simulink model "Modele_thermique"  (R2019b)
settings: Solver=FixedStepAuto  StartTime=0.0  StopTime=10.0  FixedStep=.01  RelTol=1e-3
values from neighbouring files (symbols this model uses):
  g = 9.81    [init.m]
  MOT = CBR    [init.m]
  passage_rapport = [1 2 3 4 5 6]    [init.m]
  rapport_max = 3    [init.m]
  ROUE = R13H    [init.m]
  t_passage = 0.1    [init.m]
  v_passage = [0 62.7 80.5 95 107.9 118.3]/3.6    [init.m]
undefined symbols (not defined in the file or in its folder): AERO, TRANS, VEH
libraries: simulink x1
settings Model: Creator=guillaume  LastModifiedBy=guillaume

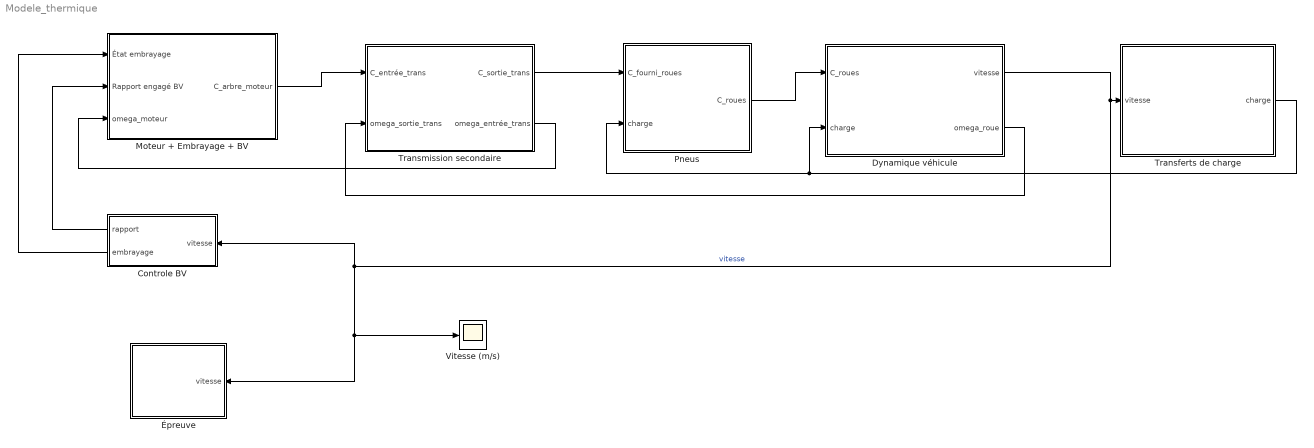
== system Modele_thermique ==
  Controle BV : Subsystem
  Dynamique véhicule : Subsystem
  Moteur + Embrayage + BV : Subsystem
  Pneus : Subsystem
  Transferts de charge : Subsystem
  Transmission secondaire : Subsystem
  Vitesse (m/s) : Scope
  Épreuve : Subsystem
  wires:
  Moteur + Embrayage + BV/1(C_arbre_moteur) -> Transmission secondaire/1(C_entrée_trans)
  Transmission secondaire/1(C_sortie_trans) -> Pneus/1(C_fourni_roues)
  Pneus/1(C_roues) -> Dynamique véhicule/1(C_roues)
  Transferts de charge/1(charge) -> Dynamique véhicule/2(charge), Pneus/2(charge)
  Dynamique véhicule/2(omega_roue) -> Transmission secondaire/2(omega_sortie_trans)
  Transmission secondaire/2(omega_entrée_trans) -> Moteur + Embrayage + BV/3(omega_moteur)
  Controle BV/1(rapport) -> Moteur + Embrayage + BV/2(Rapport engagé BV)
  Controle BV/2(embrayage) -> Moteur + Embrayage + BV/1("État embrayage ")
  Dynamique véhicule/1(vitesse) -> Controle BV/1(vitesse), Vitesse (m/s)/1, Épreuve/1(vitesse), Transferts de charge/1(vitesse)  "vitesse"

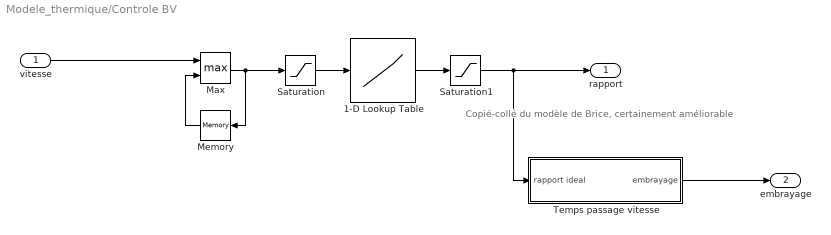
== system Modele_thermique/Controle BV ==
  note: Copié-collé du modèle de Brice, certainement améliorable
  vitesse : Inport
  1-D Lookup Table : Lookup_n-D  NumberOfTableDimensions=1  BreakpointsForDimension1=v_passage  IndexSearchMethod=Linear search  Table=passage_rapport  InterpMethod=Flat  DiagnosticForOutOfRangeInput=Warning  InternalRulePriority=Speed  OutMax=[3]  OutDataTypeStr=Inherit: Inherit from 'Table data'  RndMeth=Simplest  InputSameDT=on
  Max : MinMax  Function=max  Inputs=2
  Memory : Memory
  Saturation : Saturate  UpperLimit=inf  LowerLimit=0
  Saturation1 : Saturate  UpperLimit=rapport_max  LowerLimit=1
  "Temps passage vitesse " : Subsystem
  rapport : Outport
  embrayage : Outport  Port=2
  wires:
  vitesse/1 -> Max/1
  Max/1 -> Saturation/1, Memory/1
  Memory/1 -> Max/2
  Saturation/1 -> 1-D Lookup Table/1
  1-D Lookup Table/1 -> Saturation1/1
  "Temps passage vitesse "/1(embrayage) -> embrayage/1
  Saturation1/1 -> "Temps passage vitesse "/1(rapport ideal), rapport/1

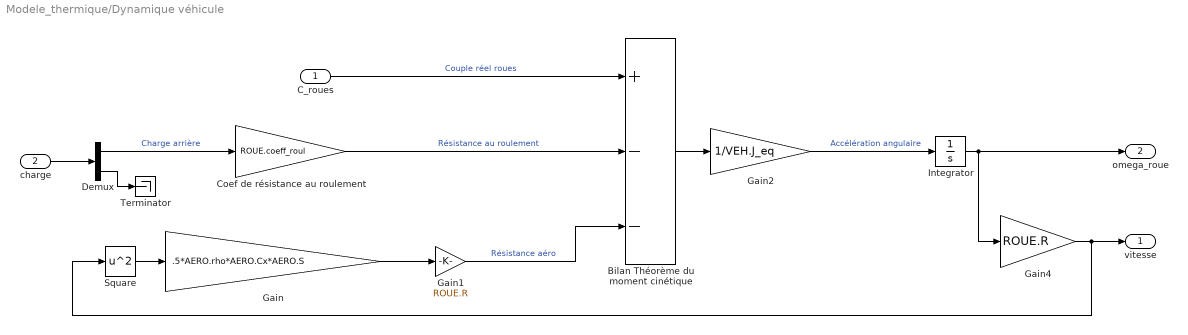
== system Modele_thermique/Dynamique véhicule ==
  C_roues : Inport
  charge : Inport  Port=2
  Bilan Théorème du moment cinétique : Sum  Inputs=+--
  Coef de résistance au roulement : Gain  Gain=ROUE.coeff_roul
  Demux : Demux  Outputs=2
  Gain : Gain  Gain=.5*AERO.rho*AERO.Cx*AERO.S
  Gain1 : Gain  Gain=ROUE.R
  Gain2 : Gain  Gain=1/VEH.J_eq
  Gain4 : Gain  Gain=ROUE.R
  Integrator : Integrator
  Square : Math  Operator=square  SignedPower=off  SaturateOnIntegerOverflow=on
  Terminator : Terminator
  vitesse : Outport
  omega_roue : Outport  Port=2
  wires:
  C_roues/1 -> Bilan Théorème du moment cinétique/1  "Couple réel roues"
  charge/1 -> Demux/1
  Demux/1 -> Coef de résistance au roulement/1  "Charge arrière"
  Coef de résistance au roulement/1 -> Bilan Théorème du moment cinétique/2  "Résistance au roulement"
  Square/1 -> Gain/1
  Gain/1 -> Gain1/1
  Gain1/1 -> Bilan Théorème du moment cinétique/3  "Résistance aéro"
  Bilan Théorème du moment cinétique/1 -> Gain2/1
  Gain2/1 -> Integrator/1  "Accélération angulaire"
  Integrator/1 -> omega_roue/1, Gain4/1
  Demux/2 -> Terminator/1
  Gain4/1 -> Square/1, vitesse/1

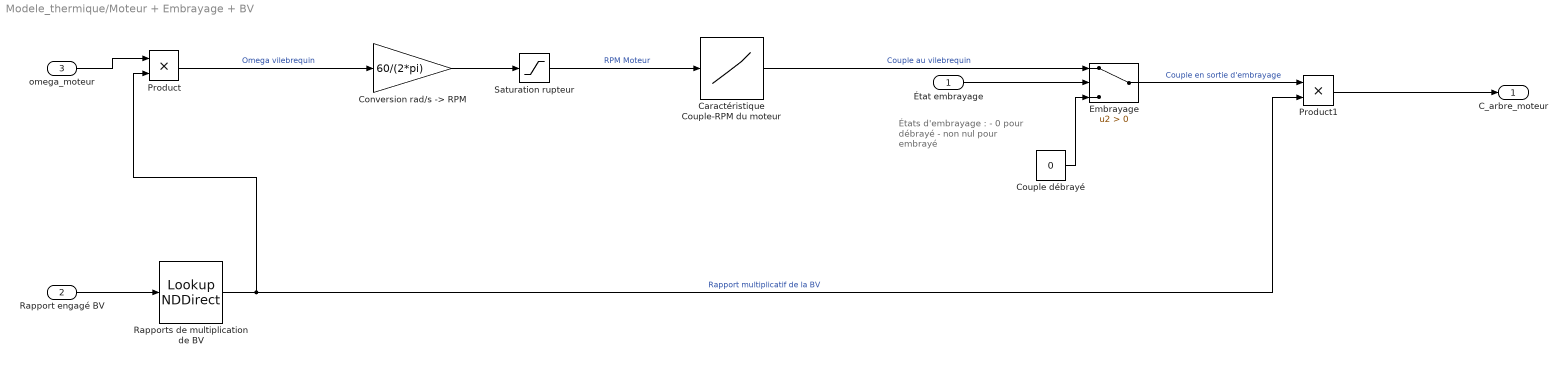
== system Modele_thermique/Moteur + Embrayage + BV ==
  note: États d'embrayage :
      | - 0 pour débrayé
      | - non nul pour embrayé
  "État embrayage " : Inport
  Rapport engagé BV : Inport  Port=2
  omega_moteur : Inport  Port=3
  Caractéristique Couple-RPM du moteur : Lookup_n-D  NumberOfTableDimensions=1  BreakpointsForDimension1=MOT.couple_RPM  Table=MOT.couple  InternalRulePriority=Speed  RndMeth=Simplest  InputSameDT=on
  "Conversion rad/s -> RPM" : Gain  Gain=60/(2*pi)
  Couple débrayé : Constant  Value=0
  Embrayage : Switch  Criteria=u2 > Threshold
  Product : Product
  Product1 : Product
  Rapports de multiplication de BV : LookupNDDirect  NumberOfTableDimensions=1  Table=[0 1./MOT.BV_rapports]  DiagnosticForOutOfRangeInput=Error
  Saturation rupteur : Saturate  UpperLimit=MOT.RPM_rupteur  LowerLimit=MOT.RPM_patinage
  C_arbre_moteur : Outport
  wires:
  Saturation rupteur/1 -> Caractéristique Couple-RPM du moteur/1  "RPM Moteur"
  Caractéristique Couple-RPM du moteur/1 -> Embrayage/1  "Couple au vilebrequin"
  Couple débrayé/1 -> Embrayage/3
  "État embrayage "/1 -> Embrayage/2
  Rapport engagé BV/1 -> Rapports de multiplication de BV/1
  Rapports de multiplication de BV/1 -> Product1/2, Product/2  "Rapport multiplicatif de la BV"
  Embrayage/1 -> Product1/1  "Couple en sortie d'embrayage"
  Product1/1 -> C_arbre_moteur/1
  "Conversion rad/s -> RPM"/1 -> Saturation rupteur/1
  Product/1 -> "Conversion rad/s -> RPM"/1  "Omega vilebrequin"
  omega_moteur/1 -> Product/1

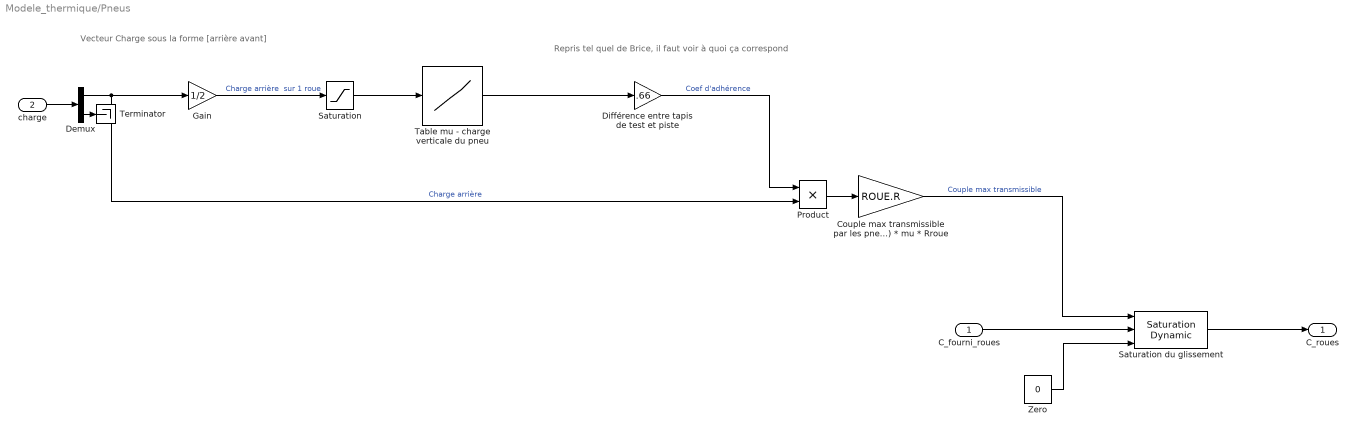
== system Modele_thermique/Pneus ==
  note: Repris tel quel de Brice,
      | il faut voir à quoi ça correspond
  note: Vecteur Charge sous la forme [arrière avant]
  C_fourni_roues : Inport
  charge : Inport  Port=2
  Couple max transmissible par les pneu chargés (2) * mu * Rroue : Gain  Gain=ROUE.R
  Demux : Demux  Outputs=2
  Différence entre tapis de test et piste : Gain  Gain=.66
  Gain : Gain  Gain=1/2
  Product : Product
  Saturation : Saturate  UpperLimit=ROUE.mupneu(1, end)  LowerLimit=ROUE.mupneu(1,1)
  Saturation du glissement : simulink/Discontinuities/Saturation Dynamic  OutMin=[0]  OutMax=[]  OutDataTypeStr=Inherit: Same as second input  OutDataType=fixdt(1, 16)  OutScaling=2^-10  DoSatur=off
  Table mu - charge verticale du pneu : Lookup_n-D  NumberOfTableDimensions=1  BreakpointsForDimension1=ROUE.mupneu(1,:)  Table=ROUE.mupneu(2,:)  DiagnosticForOutOfRangeInput=Error  InternalRulePriority=Speed  RndMeth=Simplest  InputSameDT=on
  Terminator : Terminator
  Zero : Constant  Value=0  OutDataTypeStr=Inherit: Inherit via back propagation
  C_roues : Outport
  wires:
  Saturation du glissement/1 -> C_roues/1
  Couple max transmissible par les pneu chargés (2) * mu * Rroue/1 -> Saturation du glissement/1  "Couple max transmissible"
  C_fourni_roues/1 -> Saturation du glissement/2
  charge/1 -> Demux/1
  Demux/1 -> Gain/1, Product/2  "Charge arrière"
  Table mu - charge verticale du pneu/1 -> Différence entre tapis de test et piste/1
  Différence entre tapis de test et piste/1 -> Product/1  "Coef d'adhérence"
  Product/1 -> Couple max transmissible par les pneu chargés (2) * mu * Rroue/1
  Gain/1 -> Saturation/1  "Charge arrière  sur 1 roue"
  Saturation/1 -> Table mu - charge verticale du pneu/1
  Demux/2 -> Terminator/1
  Zero/1 -> Saturation du glissement/3

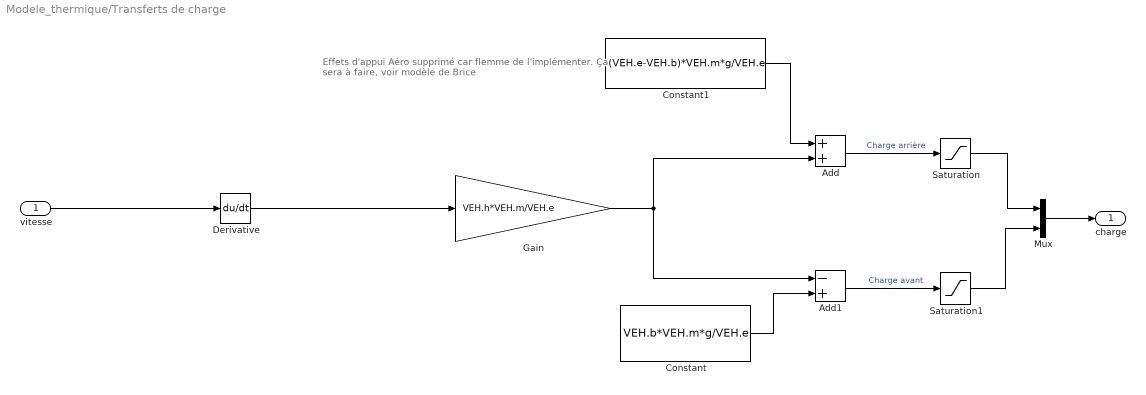
== system Modele_thermique/Transferts de charge ==
  note: Effets d'appui Aéro supprimé car flemme de l'implémenter.
      | Ça sera à faire, voir modèle de Brice
  vitesse : Inport
  Add : Sum
  Add1 : Sum  Inputs=-+
  Constant : Constant  Value=VEH.b*VEH.m*g/VEH.e
  Constant1 : Constant  Value=(VEH.e-VEH.b)*VEH.m*g/VEH.e
  Derivative : Derivative
  Gain : Gain  Gain=VEH.h*VEH.m/VEH.e
  Mux : Mux  Inputs=2
  Saturation : Saturate  UpperLimit=VEH.m*g  LowerLimit=0
  Saturation1 : Saturate  UpperLimit=inf  LowerLimit=0
  charge : Outport
  wires:
  vitesse/1 -> Derivative/1
  Constant/1 -> Add1/2
  Gain/1 -> Add/2, Add1/1
  Constant1/1 -> Add/1
  Add/1 -> Saturation/1  "Charge arrière"
  Mux/1 -> charge/1
  Saturation/1 -> Mux/1
  Saturation1/1 -> Mux/2
  Add1/1 -> Saturation1/1  "Charge avant"
  Derivative/1 -> Gain/1

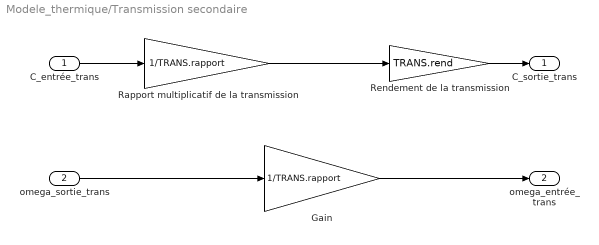
== system Modele_thermique/Transmission secondaire ==
  C_entrée_trans : Inport
  omega_sortie_trans : Inport  Port=2
  Gain : Gain  Gain=1/TRANS.rapport
  Rapport multiplicatif de la transmission : Gain  Gain=1/TRANS.rapport
  Rendement de la transmission : Gain  Gain=TRANS.rend
  C_sortie_trans : Outport
  omega_entrée_trans : Outport  Port=2
  wires:
  C_entrée_trans/1 -> Rapport multiplicatif de la transmission/1
  Rapport multiplicatif de la transmission/1 -> Rendement de la transmission/1
  Rendement de la transmission/1 -> C_sortie_trans/1
  Gain/1 -> omega_entrée_trans/1
  omega_sortie_trans/1 -> Gain/1

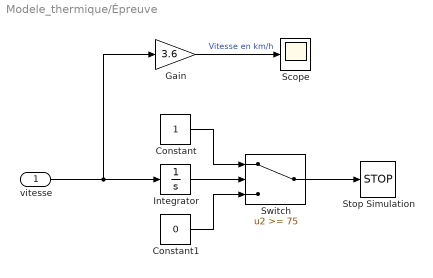
== system Modele_thermique/Épreuve ==
  vitesse : Inport
  Constant : Constant
  Constant1 : Constant  Value=0
  Gain : Gain  Gain=3.6
  Integrator : Integrator
  Scope : Scope
  Stop Simulation : Stop
  Switch : Switch  Threshold=75
  wires:
  Gain/1 -> Scope/1  "Vitesse en km/h"
  vitesse/1 -> Integrator/1, Gain/1
  Integrator/1 -> Switch/2
  Switch/1 -> Stop Simulation/1
  Constant/1 -> Switch/1
  Constant1/1 -> Switch/3

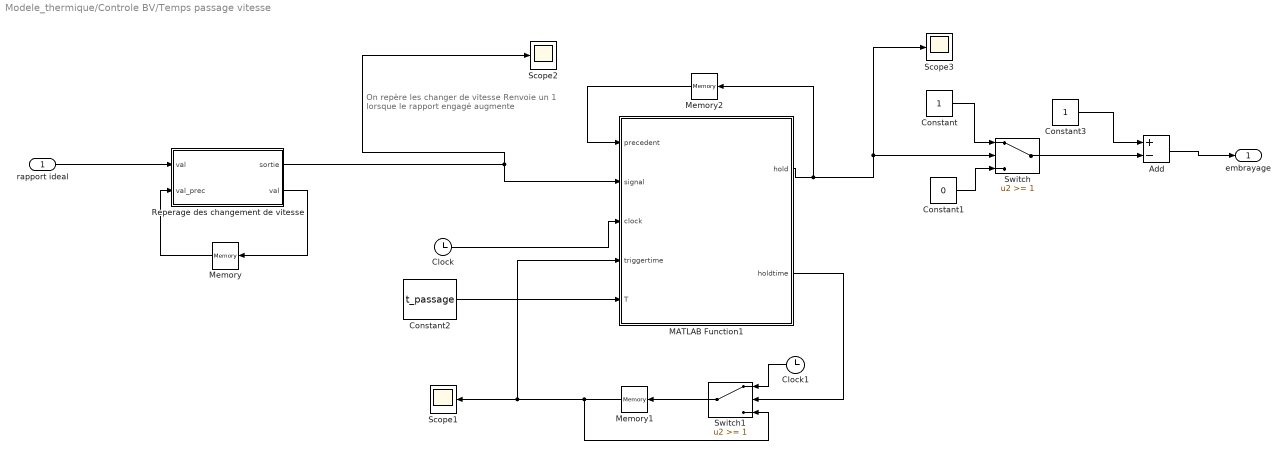
== system Modele_thermique/Controle BV/Temps passage vitesse  ==
  note: On repère les changer de vitesse
      | Renvoie un 1 lorsque le rapport engagé augmente
  rapport ideal : Inport
  Add : Sum  Inputs=+-
  Clock : Clock
  Clock1 : Clock
  Constant : Constant
  Constant1 : Constant  Value=0
  Constant2 : Constant  Value=t_passage
  Constant3 : Constant
  MATLAB Function1 : MATLAB Function  TreatAsAtomicUnit=on
  Memory : Memory  InitialCondition=1
  Memory1 : Memory
  Memory2 : Memory
  Reperage des changement de vitesse : MATLAB Function  TreatAsAtomicUnit=on
  Scope1 : Scope
  Scope2 : Scope
  Scope3 : Scope
  Switch : Switch  Threshold=1
  Switch1 : Switch  Threshold=1
  embrayage : Outport
  wires:
  rapport ideal/1 -> Reperage des changement de vitesse/1("val ")
  Memory/1 -> Reperage des changement de vitesse/2(val_prec)
  Reperage des changement de vitesse/2(val) -> Memory/1
  Reperage des changement de vitesse/1(sortie) -> Scope2/1, MATLAB Function1/2(signal)
  MATLAB Function1/1(hold) -> Scope3/1, Switch/2, Memory2/1
  Switch1/1 -> Memory1/1
  MATLAB Function1/2(holdtime) -> Switch1/2
  Constant/1 -> Switch/1
  Constant1/1 -> Switch/3
  Memory1/1 -> Switch1/3, MATLAB Function1/4(triggertime), Scope1/1
  Memory2/1 -> MATLAB Function1/1(precedent)
  Clock1/1 -> Switch1/1
  Clock/1 -> MATLAB Function1/3(clock)
  Constant2/1 -> MATLAB Function1/5(T)
  Switch/1 -> Add/2
  Add/1 -> embrayage/1
  Constant3/1 -> Add/1

== matlab function Modele_thermique/Controle BV/Temps passage vitesse /MATLAB Function1 ==
  data: precedent input; hold output; holdtime output; signal input; clock input; triggertime input; T input
function [hold, holdtime]= fcn(precedent, signal, clock, triggertime, T)
%#Si on repère un changement de rapport, alors on crée un signal créneau ayant la valeur 1 pendant une durée de t_passage

hold = 0;
holdtime = 0;


if signal == 1
    hold = 1;
    holdtime = 1;
end

if precedent == 1 && clock < triggertime + T
    hold = 1;
    holdtime = 0;
end
end

== matlab function Modele_thermique/Controle BV/Temps passage vitesse /Reperage des changement de vitesse ==
  data: val input; sortie output; val_prec input; val output
function [sortie, val]= fcn(val, val_prec)
%#Cette fonction renvoie 1 lorsque l'on change de vitesse
if val == val_prec
    sortie = 0;
else
    sortie = 1;
end
